simulink model "functions_blocks"  (R2025a)
settings: Solver=VariableStepAuto  StartTime=0.0  StopTime=0.01  RelTol=1e-3
libraries: phasedwavlib x1
settings Model: Creator=Admin  LastModifiedBy=Admin

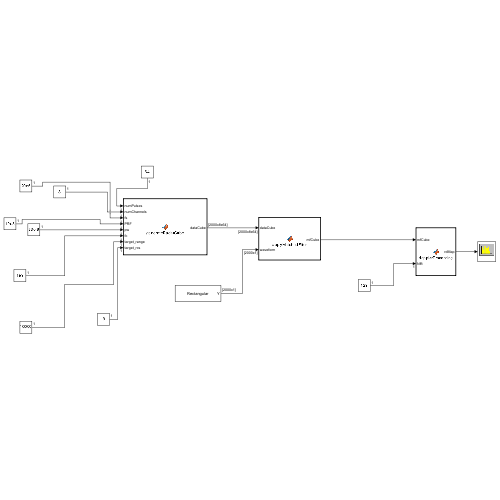
[thumbnail: Simulink's stored preview of the top-level diagram]
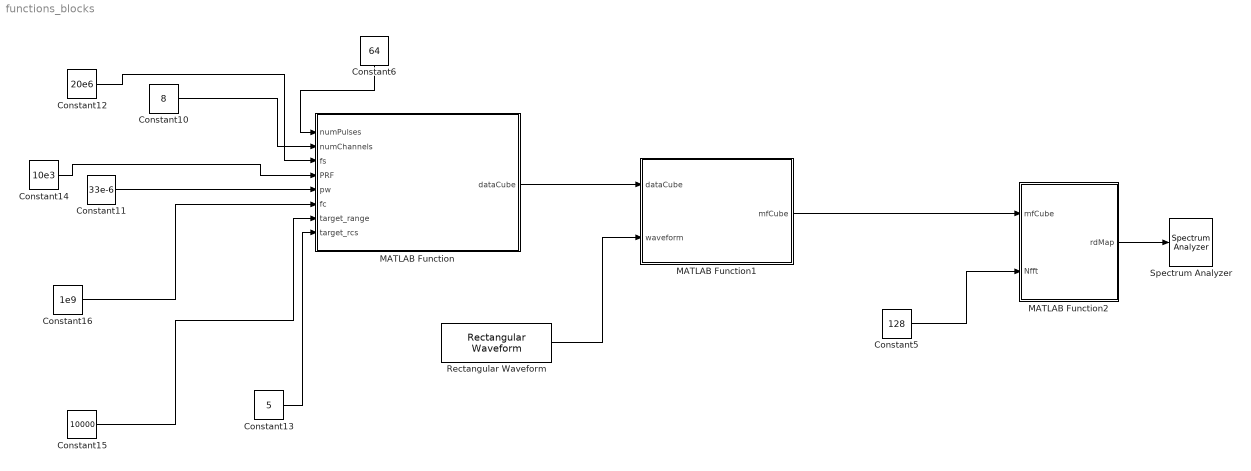
== system functions_blocks ==
  Constant10 : Constant  Value=8
  Constant11 : Constant  Value=33e-6
  Constant12 : Constant  Value=20e6
  Constant13 : Constant  Value=5
  Constant14 : Constant  Value=10e3
  Constant15 : Constant  Value=10000
  Constant16 : Constant  Value=1e9
  Constant5 : Constant  Value=128
  Constant6 : Constant  Value=64
  MATLAB Function : MATLAB Function  TreatAsAtomicUnit=on
  MATLAB Function1 : MATLAB Function  TreatAsAtomicUnit=on
  MATLAB Function2 : MATLAB Function  TreatAsAtomicUnit=on
  Rectangular Waveform : phasedwavlib/Rectangular Waveform  SampleRate=20e6  DurationSpecification=Pulse width  PulseWidth=33e-6  DutyCycle=0.5  PRF=1e4  PRFSelectionInputPort=off  SimulationTimeSource=Derive from waveform parameters  FrequencyOffsetSource=Property  FrequencyOffset=0  OutputFormat=Pulses  NumSamples=100  NumPulses=1  PRFOutputPort=off  CoefficientsOutputPort=off  SimulateUsing=Interpreted execution
  Spectrum Analyzer : SpectrumAnalyzer  WindowInvariantSamplesPerUpdate=on
  wires:
  MATLAB Function/1(dataCube) -> MATLAB Function1/1(dataCube)
  MATLAB Function1/1(mfCube) -> MATLAB Function2/1(mfCube)
  Constant13/1 -> MATLAB Function/8(target_rcs)
  Constant15/1 -> MATLAB Function/7(target_range)
  Constant16/1 -> MATLAB Function/6(fc)
  Constant11/1 -> MATLAB Function/5(pw)
  Constant14/1 -> MATLAB Function/4(PRF)
  Constant6/1 -> MATLAB Function/1(numPulses)
  Constant10/1 -> MATLAB Function/2(numChannels)
  Constant12/1 -> MATLAB Function/3(fs)
  Rectangular Waveform/1 -> MATLAB Function1/2(waveform)
  Constant5/1 -> MATLAB Function2/2(Nfft)
  MATLAB Function2/1(rdMap) -> Spectrum Analyzer/1

== matlab function functions_blocks/MATLAB Function1 ==
  data: dataCube input; mfCube output; waveform input
function mfCube = applyMatchedFilter(dataCube,waveform)
    ref = getMatchedFilter(waveform);
    [N,K,L] = size(dataCube);
    mfCube = zeros(N,K,L);
    for ch = 1:L
        for p = 1:K
            mfCube(:,p,ch) = conv(dataCube(:,p,ch),ref,'same');
        end
    end
end

== matlab function functions_blocks/MATLAB Function ==
  data: numPulses input; dataCube output double size=2000 8 64; numChannels input; fs input; PRF input; pw input; fc input; target_range input; target_rcs input
function dataCube = generateRadarCube(numPulses,numChannels,fs,PRF,pw,fc,target_range,target_rcs)
    % Radar waveform
    waveform = phased.RectangularWaveform('SampleRate',fs,'PRF',PRF,'PulseWidth',pw);
    
    % Array
    C = physconst('LightSpeed');
    antenna = phased.IsotropicAntennaElement('FrequencyRange',[800e6 1.2e9]);
    Array = phased.ULA('NumElements',numChannels,'ElementSpacing',0.5*(C/fc),'Element',antenna);
    
    % Transmitter
    transmitter = phased.Transmitter('Gain',20,'PeakPower',5000);
    
    % Target
    target = phased.RadarTarget('MeanRCS',target_rcs,'OperatingFrequency',fc);
    
    % Free space channel
    channel = phased.FreeSpace('SampleRate',fs,'TwoWayPropagation',false,'OperatingFrequency',fc);
    
    % Collector & Receiver
    collector = phased.Collector('Sensor',Array,'OperatingFrequency',fc);
    receiver  = phased.ReceiverPreamp('Gain',0,'NoiseFigure',10,'SampleRate',fs);
    
    % Sizes
    samplesPerPulse = round(fs/PRF);
    dataCube = complex(zeros(samplesPerPulse,numPulses,numChannels));   
    % Positions
    radarPos = [0;0;0]; radarVel = [0;0;0];
    targetPos = [target_range;0;0]; targetVel = [0;0;0];
    
    % Loop pulses
    for p = 1:numPulses
        sig = waveform();
        txsig = transmitter(sig);
        propsig = channel(txsig,radarPos,targetPos,radarVel,targetVel);
        reflsig = target(propsig);
        rxsig  = channel(reflsig,targetPos,radarPos,targetVel,radarVel);
        rxsig  = collector(rxsig,[0;0]);
        rxsig  = receiver(rxsig);
        
        dataCube(:,p,:) = rxsig(1:samplesPerPulse,:);
    end
end

== matlab function functions_blocks/MATLAB Function2 ==
  data: mfCube input; rdMap output; Nfft input
function rdMap = dopplerProcessing(mfCube,Nfft)
    % Take one channel for now
    rdMap = fftshift(fft(mfCube(:,:,1),Nfft,2),2);
end
